simulink model "example_main_NDI_f16"  (R2020a)
settings: Solver=ode4  StartTime=0.0  StopTime=75  FixedStep=0.01  RelTol=1e-3
PreLoadFcn:
  | PreLoadFcn
values from neighbouring files (symbols this model uses):
  g = 32.17    [PreLoadFcn.m]
  N = [ 1      0     0.25 ... (first row only)    [PreLoadFcn.m]
  state0 = [IC.npos IC.epos IC.alt IC.q0 IC.q1 IC.q2 IC.q3  IC.p IC.q IC.r IC.alpha IC.beta IC.mu IC.Vt IC.chi IC.gamma]    [PreLoadFcn.m]
undefined symbols (not defined in the file or in its folder): Aactuator, ac, AeroCoeff, EngineTable, ft, IC, kg, m, Newton, PIController, Raphson, s, sigbuilder_block, slug
libraries: aerolibconvert2 x19, simulink x13, sharedutil x1
(part 4 of 6)

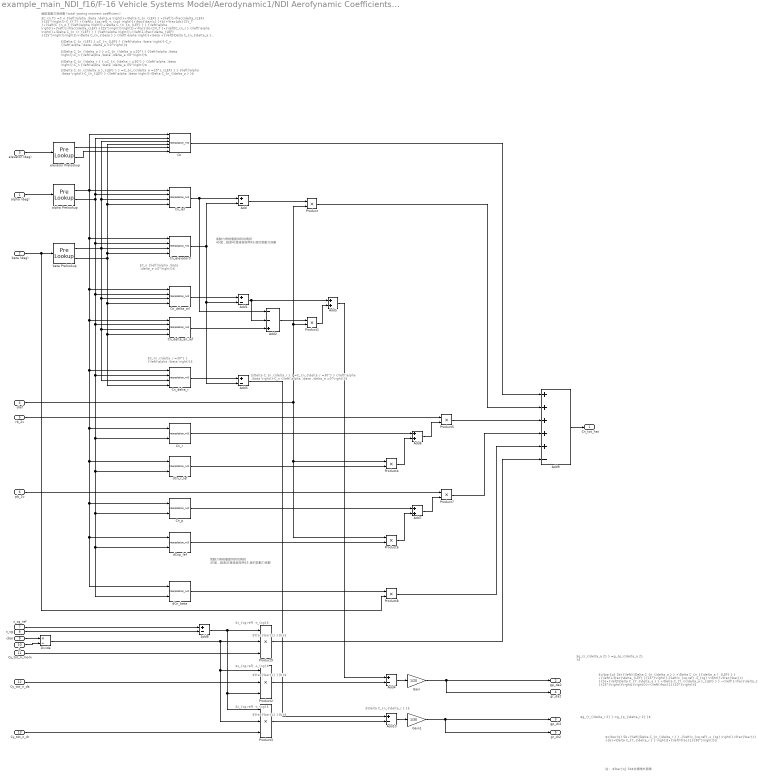
== system example_main_NDI_f16/F-16 Vehicle Systems Model/Aerodynamic1/NDI Aerofynamic Coefficients/CnT ==
  note: $C_n {\left(\alpha ,\beta ,\delta_e =0°\right)}$
  note: $C_{n_{\delta_r =30°} } {\left(\alpha ,\beta \right)}$
  note: $\Delta C_{n_{\delta_r } } =C_{n_{\delta_r =30°} } {\left(\alpha ,\beta \right)}-C_n {\left(\alpha ,\beta ,\delta_e =0°\right)}$
  note: $\Delta C_{n_{\delta_r } }$
  note: $\frac{\bar{c} }{b}$
  note: $x_{cg,ref} -x_{cg}$
  note: 註： $\bar{q} Sb$ 在模塊外面乘
  note: $=\bar{q} Sb∙{\left\{\Delta C_{n_{\delta_a } } +\Delta C_{n_{{\delta_a }_{LEF} } } ∙{\left(1-\frac{\delta_{LEF} }{25°}\right)}-{\left(x_{cg,ref} -x_{cg} \right)}∙\frac{\bar{c} }{b}∙{\left[\Delta C_{Y_{\delta_a } } +\Delta C_{Y_{{\delta_a }_{LEF} } } ∙{\left(1-\frac{\delta_{LEF} }{25°}\right)}\right]}\right\}}∙{\left(\frac{1}{20°}\right)}$
  note: $g_{r_{\delta_a 2} } =g_{p_{\delta_a 2} }$
  note: $=\bar{q} Sb∙{\left[\Delta C_{n_{\delta_r } } -{\left(x_{cg,ref} -x_{cg} \right)}∙\frac{\bar{c} }{b}∙\Delta C_{Y_{\delta_r } } \right]}∙{\left(\frac{1}{30°}\right)}$
  note: $g_{r_{\delta_r 2} } =g_{p_{\delta_r 2} }$
  note: 氣動力表格僅提供到攻角到
      | 45度，超過45度後皆採用45
      | 度的氣動力係數
  note: 氣動力表格僅提供到攻角到
      | 45度，超過45度後皆採用45
      | 度的氣動力係數
  note: $x_{cg,ref} -x_{cg}$
  note: $x_{cg,ref} -x_{cg}$
  note: $\frac{\bar{c} }{b}$
  note: $\frac{\bar{c} }{b}$
  note: $\Delta C_{n_{LEF} } =C_{n_{LEF} } {\left(\alpha ,\beta \right)}-C_n {\left(\alpha ,\beta ,\delta_e =0°\right)}$
  note: 偏航氣動力矩係數 (total yawing moment coefficient)：
  note: $\Delta C_{n_{\delta_a } } =C_{n_{\delta_a =20°} } {\left(\alpha ,\beta \right)}-C_n {\left(\alpha ,\beta ,\delta_e =0°\right)}$
  note: $\Delta C_{n_{\delta_r } } =C_{n_{\delta_r =30°} } {\left(\alpha ,\beta \right)}-C_n {\left(\alpha ,\beta ,\delta_e =0°\right)}$
  note: $\Delta C_{n_{{\delta_a }_{LEF} } } =C_{n_{{\delta_a =20°}_{LEF} } } {\left(\alpha ,\beta \right)}-C_{n_{LEF} } {\left(\alpha ,\beta \right)}-\Delta C_{n_{\delta_a } }$
  note: $C_{n,T} =C_n {\left(\alpha ,\beta ,\delta_e \right)}+\Delta C_{n_{LEF} } ∙{\left(1-\frac{\delta_{LEF} }{25°}\right)}-C_{Y,T} ∙{\left(x_{cg,ref} -x_{cg} \right)}∙\frac{\bar{c} }{b}+\frac{pb}{2V_T }∙{\left[C_{n_p } {\left(\alpha \right)}+\Delta C_{n_{p_{LEF} } } {\left(\alpha \right)}∙{\left(1-\frac{\delta_{LEF} }{25°}\right)}\right]}+\frac{rb}{2V_T }∙{\left[C_{n_r } {\left(\alpha \right)}+\Delta C_{n_{r_{LEF} } } {\left(\alpha \right)}∙{\left(1-\frac{\delta_{LEF} }{25°}\right)}\right]}+\Delta C_{n_{\beta } } {\left(\alpha \right)}∙\beta +{\left[\Delta C_{n_{\delta_a } } +\Delta C_{n_{{\delta_a }_{LEF} } } ∙{\left(1-\frac{\delta_{LEF} }{25°}\right)}\right]}∙{\left(\frac{\delta_a }{20°}\right)}+\Delta C_{n_{\delta_r } } ∙{\left(\frac{\delta_r }{30°}\right)}$
  alpha (deg) : Inport
  beta (deg) : Inport  Port=2
  elevator (deg) : Inport  Port=3
  dlef : Inport  Port=4
  rb_2v : Inport  Port=5
  pb_2v : Inport  Port=6
  x_cg_ref : Inport  Port=7
  x_cg : Inport  Port=8
  cbar : Inport  Port=9
  b : Inport  Port=10
  Cy_tot_n_mom : Inport  Port=11
  Cy_tot_n_da : Inport  Port=12
  Cy_tot_n_dr : Inport  Port=13
  Add{,1,3..4,8,10} (6 alike) : Sum  Inputs=+-
  Add2 : Sum  Inputs=--+
  Add5 : Sum
  Add6 : Sum
  Add7 : Sum
  Add9 : Sum  Inputs=+++++-
  Cn : Interpolation_n-D  NumberOfTableDimensions=3  Table=AeroCoeff.Cn
      settings: InputPortMap=u0,u1,u2,u3,u4,u5
  Cn_delta_ail : Interpolation_n-D  Table=AeroCoeff.Cn_delta_ail
  Cn_delta_ail_lef : Interpolation_n-D  Table=AeroCoeff.Cn_delta_ail_lef
  Cn_delta_r : Interpolation_n-D  Table=AeroCoeff.Cn_delta_r
  Cn_elevator0 : Interpolation_n-D  Table=AeroCoeff.Cn_elevator0
  Cn_lef : Interpolation_n-D  Table=AeroCoeff.Cn_lef
  Cn_p : Interpolation_n-D  NumberOfTableDimensions=1  Table=AeroCoeff.Cn_p
      settings: InputPortMap=u0,u1
  Cn_r : Interpolation_n-D  NumberOfTableDimensions=1  Table=AeroCoeff.Cn_r
      settings: InputPortMap=u0,u1
  Divide : Product  Inputs=*/
  Gain : Gain  Gain=1/20
  Gain1 : Gain  Gain=1/30
  Product{,1,4..8} (7 alike) : Product
  Product2 : Product  Inputs=3
  Product3 : Product  Inputs=3
  Product9 : Product  Inputs=3
  alpha Prelookup : PreLookup  BreakpointsData=AeroCoeff.alpha_prelookup  IndexSearchMethod=Linear search  BeginIndexSearchUsingPreviousIndexResult=on  DiagnosticForOutOfRangeInput=Warning
  beta Prelookup : PreLookup  BreakpointsData=AeroCoeff.beta_prelookup  IndexSearchMethod=Linear search  BeginIndexSearchUsingPreviousIndexResult=on  DiagnosticForOutOfRangeInput=Warning
  dCn_beta : Interpolation_n-D  NumberOfTableDimensions=1  Table=AeroCoeff.dCn_beta
      settings: InputPortMap=u0,u1
  dCn_r_lef : Interpolation_n-D  NumberOfTableDimensions=1  Table=AeroCoeff.dCn_r_lef
      settings: InputPortMap=u0,u1
  dCnp_lef : Interpolation_n-D  NumberOfTableDimensions=1  Table=AeroCoeff.dCnp_lef
      settings: InputPortMap=u0,u1
  elevator Prelookup : PreLookup  BreakpointsData=AeroCoeff.elevator_prelookup1  IndexSearchMethod=Linear search  BeginIndexSearchUsingPreviousIndexResult=on  DiagnosticForOutOfRangeInput=Warning
  Cn_tot_hat : Outport  VectorParamsAs1DForOutWhenUnconnected=off
  gp_da2 : Outport  Port=2  VectorParamsAs1DForOutWhenUnconnected=off
  gp_dr2 : Outport  Port=3  VectorParamsAs1DForOutWhenUnconnected=off
  gr_da2 : Outport  Port=4  VectorParamsAs1DForOutWhenUnconnected=off
  gr_dr2 : Outport  Port=5  VectorParamsAs1DForOutWhenUnconnected=off
  wires:
  alpha Prelookup/1 -> Cn_r/1, dCn_beta/1, dCnp_lef/1, Cn_p/1, dCn_r_lef/1, Cn_delta_r/1, Cn_delta_ail_lef/1, Cn_delta_ail/1, Cn_elevator0/1, Cn/1, Cn_lef/1
  Add8/1 -> Product3/1, Product2/3, Product9/1
  Add1/1 -> Add2/2, Add5/1
  Cn_elevator0/1 -> Add/2, Add3/2, Add1/2
  alpha Prelookup/2 -> Cn_r/2, dCn_beta/2, dCnp_lef/2, Cn_p/2, dCn_r_lef/2, Cn_delta_r/2, Cn_delta_ail_lef/2, Cn_delta_ail/2, Cn_elevator0/2, Cn/2, Cn_lef/2
  elevator Prelookup/1 -> Cn/5
  Add6/1 -> Product5/2
  beta Prelookup/2 -> Cn/4, Cn_lef/4, Cn_elevator0/4, Cn_delta_r/4, Cn_delta_ail_lef/4, Cn_delta_ail/4
  Cn_r/1 -> Add6/1
  Cn_delta_ail_lef/1 -> Add2/3
  pb_2v/1 -> Product7/1
  Cn_lef/1 -> Add2/1, Add/1
  Add7/1 -> Product7/2
  beta (deg)/1 -> beta Prelookup/1, Product8/2
  rb_2v/1 -> Product5/1
  Add/1 -> Product/1
  x_cg/1 -> Add8/2
  alpha (deg)/1 -> alpha Prelookup/1
  b/1 -> Divide/2
  dCn_r_lef/1 -> Product4/2
  dCn_beta/1 -> Product8/1
  Product4/1 -> Add6/2
  Divide/1 -> Product3/2, Product2/1, Product9/2
  x_cg_ref/1 -> Add8/1
  Cn_p/1 -> Add7/1
  dCnp_lef/1 -> Product6/2
  Product8/1 -> Add9/5
  elevator Prelookup/2 -> Cn/6
  Cn_delta_r/1 -> Add3/1
  Product6/1 -> Add7/2
  Cy_tot_n_mom/1 -> Product9/3
  Product7/1 -> Add9/4
  Product5/1 -> Add9/3
  Add2/1 -> Product1/1
  beta Prelookup/1 -> Cn/3, Cn_lef/3, Cn_delta_r/3, Cn_delta_ail_lef/3, Cn_delta_ail/3, Cn_elevator0/3
  Cn/1 -> Add9/1
  Cn_delta_ail/1 -> Add1/1
  Add3/1 -> Add10/1
  elevator (deg)/1 -> elevator Prelookup/1
  dlef/1 -> Product4/1, Product6/1, Product/2, Product1/2
  Product/1 -> Add9/2
  Product1/1 -> Add5/2
  cbar/1 -> Divide/1
  Product9/1 -> Add9/6
  Cy_tot_n_da/1 -> Product2/2
  Product2/1 -> Add4/2
  Add5/1 -> Add4/1
  Add4/1 -> Gain/1
  Cy_tot_n_dr/1 -> Product3/3
  Product3/1 -> Add10/2
  Add10/1 -> Gain1/1
  Add9/1 -> Cn_tot_hat/1
  Gain/1 -> gr_da2/1, gp_da2/1
  Gain1/1 -> gr_dr2/1, gp_dr2/1

== system example_main_NDI_f16/F-16 Vehicle Systems Model/Aerodynamic1/NDI Aerofynamic Coefficients/Ground Effects ==
  alpha (deg) : Inport
  beta(deg) : Inport  Port=2
  h_AGL : Inport  Port=3
  Coeff : Outport

== system example_main_NDI_f16/F-16 Vehicle Systems Model/Aerodynamic1/NDI Aerofynamic Coefficients/Landing Gear Effects ==
  alpha (deg) : Inport
  beta(deg) : Inport  Port=2
  Landing Gear Angle : Inport  Port=3
  Coeff : Outport

== system example_main_NDI_f16/F-16 Vehicle Systems Model/Aerodynamic2/NDI Aerofynamic Coefficients/CXT ==
  note: 氣動力表格僅提供到攻角到
      | 45度，超過45度後皆採用45
      | 度的氣動力係數
  note: $\Delta C_{X_{LEF} } =C_{X_{LEF} } {\left(\alpha ,\beta \right)}-C_X {\left(\alpha ,\beta ,\delta_e =0°\right)}$
  note: $C_{X,T} =C_X {\left(\alpha ,\beta ,\delta_e \right)}+\Delta C_{X_{LEF} } ∙{\left(1-\frac{\delta_{LEF} }{25°}\right)}+\frac{q\bar{c} }{2V_T }∙{\left[C_{X_q } {\left(\alpha \right)}+\Delta C_{X_{q_{LEF} } } {\left(\alpha \right)}∙{\left(1-\frac{\delta_{LEF} }{25°}\right)}\right]}+\Delta C_{X_{SB} } {\left(\alpha \right)}∙{\left(\frac{\delta_{SB} }{60°}\right)}$
  note: 體軸 x 方向之氣動力係數 (total x-axis force coefficient)：
  alpha (deg) : Inport
  beta (deg) : Inport  Port=2
  elevator (deg) : Inport  Port=3
  dlef : Inport  Port=4
  qc_2v : Inport  Port=5
  sb : Inport  Port=6
  Add : Sum  Inputs=+-
  Add1 : Sum  Inputs=++++
  Add2 : Sum
  Cx : Interpolation_n-D  NumberOfTableDimensions=3  Table=AeroCoeff.Cx
      settings: InputPortMap=u0,u1,u2,u3,u4,u5
  Cx_elevator0 : Interpolation_n-D  Table=AeroCoeff.Cx_elevator0
  Cx_lef : Interpolation_n-D  Table=AeroCoeff.Cx_lef
  Cx_q : Interpolation_n-D  NumberOfTableDimensions=1  Table=AeroCoeff.Cx_q
      settings: InputPortMap=u0,u1
  Cx_q_lef : Interpolation_n-D  NumberOfTableDimensions=1  Table=AeroCoeff.Cx_q_lef
      settings: InputPortMap=u0,u1
  Product{,1..3} (4 alike) : Product
  alpha Prelookup : PreLookup  BreakpointsData=AeroCoeff.alpha_prelookup  IndexSearchMethod=Linear search  BeginIndexSearchUsingPreviousIndexResult=on  DiagnosticForOutOfRangeInput=Warning
  beta Prelookup : PreLookup  BreakpointsData=AeroCoeff.beta_prelookup  IndexSearchMethod=Linear search  BeginIndexSearchUsingPreviousIndexResult=on  DiagnosticForOutOfRangeInput=Warning
  dCX_sb : Interpolation_n-D  NumberOfTableDimensions=1  Table=AeroCoeff.dCX_sb
      settings: InputPortMap=u0,u1
  elevator Prelookup : PreLookup  BreakpointsData=AeroCoeff.elevator_prelookup2  IndexSearchMethod=Linear search  BeginIndexSearchUsingPreviousIndexResult=on  DiagnosticForOutOfRangeInput=Warning
  Cx_tot : Outport  VectorParamsAs1DForOutWhenUnconnected=off
  wires:
  beta Prelookup/2 -> Cx_elevator0/4, Cx_lef/4, Cx/4
  alpha (deg)/1 -> alpha Prelookup/1
  beta Prelookup/1 -> Cx_elevator0/3, Cx_lef/3, Cx/3
  Cx_lef/1 -> Add/1
  alpha Prelookup/1 -> Cx_q_lef/1, dCX_sb/1, Cx_q/1, Cx_elevator0/1, Cx/1, Cx_lef/1
  elevator Prelookup/2 -> Cx/6
  elevator (deg)/1 -> elevator Prelookup/1
  beta (deg)/1 -> beta Prelookup/1
  Add/1 -> Product/1
  alpha Prelookup/2 -> Cx_q_lef/2, dCX_sb/2, Cx_q/2, Cx_elevator0/2, Cx_lef/2, Cx/2
  Product/1 -> Add1/2
  elevator Prelookup/1 -> Cx/5
  Add2/1 -> Product2/1
  Cx/1 -> Add1/1
  Cx_elevator0/1 -> Add/2
  Cx_q_lef/1 -> Product1/1
  Product1/1 -> Add2/2
  Cx_q/1 -> Add2/1
  dlef/1 -> Product/2, Product1/2
  Product2/1 -> Add1/3
  Add1/1 -> Cx_tot/1
  qc_2v/1 -> Product2/2
  dCX_sb/1 -> Product3/1
  sb/1 -> Product3/2
  Product3/1 -> Add1/4

== system example_main_NDI_f16/F-16 Vehicle Systems Model/Aerodynamic2/NDI Aerofynamic Coefficients/CYT ==
  note: 氣動力表格僅提供到攻角到
      | 45度，超過45度後皆採用45
      | 度的氣動力係數
  note: 氣動力表格僅提供到攻角到
      | 45度，超過45度後皆採用45
      | 度的氣動力係數
  note: 體軸 y 方向之氣動力係數 (total y-axis force coefficient)：
  note: $\Delta C_{Y_{LEF} }=C_{Y_{LEF} } {\left(\alpha ,\beta \right)}\ \ -C_Y {\left(\alpha ,\beta \right)}$
  note: $\Delta C_{Y_{\delta_r } }=C_{Y_{\delta_r =30°} } {\left(\alpha ,\beta \right)}-C_Y {\left(\alpha ,\beta \right)}$
  note: $C_{Y,T} =C_Y {\left(\alpha ,\beta \right)}+\Delta C_{Y_{LEF} } ∙{\left(1-\frac{\delta_{LEF} }{25°}\right)}+\frac{pb}{2V_T }∙{\left[C_{Y_p } {\left(\alpha \right)}+\Delta C_{{Y_p }_{LEF} } {\left(\alpha \right)}∙{\left(1-\frac{\delta_{LEF} }{25°}\right)}\right]}+\frac{rb}{2V_T }∙{\left[C_{Y_r } {\left(\alpha \right)}+\Delta C_{{Y_r }_{LEF} } {\left(\alpha \right)}∙{\left(1-\frac{\delta_{LEF} }{25°}\right)}\right]}+{\left[\Delta C_{Y_{\delta_a } } +\Delta C_{Y_{{\delta_a }_{LEF} } } ∙{\left(1-\frac{\delta_{LEF} }{25°}\right)}\right]}∙{\left(\frac{\delta_a }{20°}\right)}+\Delta C_{Y_{\delta_r } } ∙{\left(\frac{\delta_r }{30°}\right)}$
  note: $\Delta C_{Y_{{\delta_a }_{LEF} } } =C_{Y_{{\delta_a =20°}_{LEF} } } {\left(\alpha ,\beta \right)}-C_{Y_{LEF} } {\left(\alpha ,\beta \right)}-\Delta C_{Y_{\delta_a } }$
  note: $\Delta C_{Y_{\delta_a } }=C_{Y_{\delta_a =20°} } {\left(\alpha ,\beta \right)}-C_Y {\left(\alpha ,\beta \right)}$
  alpha (deg) : Inport
  beta (deg) : Inport  Port=2
  dlef : Inport  Port=3
  dail : Inport  Port=4
  drud : Inport  Port=5
  rb_2v : Inport  Port=6
  pb_2v : Inport  Port=7
  Add : Sum  Inputs=-+
  Add1 : Sum  Inputs=-+
  Add2 : Sum  Inputs=+--
  Add3 : Sum  Inputs=+-
  Add4 : Sum  Inputs=++++++
  Add5 : Sum
  Add6 : Sum
  Add7 : Sum
  Add8 : Sum  Inputs=++++
  CY : Interpolation_n-D  Table=AeroCoeff.CY
  CY_delta_ail : Interpolation_n-D  Table=AeroCoeff.CY_delta_ail
  CY_delta_ail_lef : Interpolation_n-D  Table=AeroCoeff.CY_delta_ail_lef
  CY_delta_r : Interpolation_n-D  Table=AeroCoeff.CY_delta_r
  CY_lef : Interpolation_n-D  Table=AeroCoeff.CY_lef
  CY_p : Interpolation_n-D  NumberOfTableDimensions=1  Table=AeroCoeff.CY_p
      settings: InputPortMap=u0,u1
  CY_r : Interpolation_n-D  NumberOfTableDimensions=1  Table=AeroCoeff.CY_r
      settings: InputPortMap=u0,u1
  Product{,1..7} (8 alike) : Product
  alpha Prelookup : PreLookup  BreakpointsData=AeroCoeff.alpha_prelookup  IndexSearchMethod=Linear search  BeginIndexSearchUsingPreviousIndexResult=on  DiagnosticForOutOfRangeInput=Warning
  beta Prelookup : PreLookup  BreakpointsData=AeroCoeff.beta_prelookup  IndexSearchMethod=Linear search  BeginIndexSearchUsingPreviousIndexResult=on  DiagnosticForOutOfRangeInput=Warning
  dCY_p_lef : Interpolation_n-D  NumberOfTableDimensions=1  Table=AeroCoeff.dCY_p_lef
      settings: InputPortMap=u0,u1
  dCY_r_lef : Interpolation_n-D  NumberOfTableDimensions=1  Table=AeroCoeff.dCY_r_lef
      settings: InputPortMap=u0,u1
  Cy_tot : Outport  VectorParamsAs1DForOutWhenUnconnected=off
  Cy_tot_n_mom : Outport  Port=2  VectorParamsAs1DForOutWhenUnconnected=off
  Cy_tot_n_da : Outport  Port=3  VectorParamsAs1DForOutWhenUnconnected=off
  Cy_tot_n_dr : Outport  Port=4  VectorParamsAs1DForOutWhenUnconnected=off
  wires:
  Add3/1 -> Cy_tot_n_dr/1, Product3/1
  beta Prelookup/2 -> CY_delta_r/4, CY_delta_ail_lef/4, CY_delta_ail/4, CY/4, CY_lef/4
  beta Prelookup/1 -> CY_delta_r/3, CY_delta_ail_lef/3, CY_delta_ail/3, CY/3, CY_lef/3
  Product7/1 -> Add4/6, Add8/4
  dlef/1 -> Product1/2, Product/2, Product4/2, Product6/1
  alpha Prelookup/1 -> dCY_p_lef/1, CY_p/1, dCY_r_lef/1, CY_r/1, CY_delta_r/1, CY_delta_ail_lef/1, CY_delta_ail/1, CY_lef/1, CY/1
  Add4/1 -> Cy_tot/1
  Add5/1 -> Cy_tot_n_da/1, Product2/1
  CY_p/1 -> Add7/1
  Add1/1 -> Add2/3, Add5/1
  CY_lef/1 -> Add/2, Add2/2
  Add/1 -> Product/1
  dCY_p_lef/1 -> Product6/2
  CY_delta_r/1 -> Add3/1
  CY_delta_ail_lef/1 -> Add2/1
  dCY_r_lef/1 -> Product4/1
  alpha (deg)/1 -> alpha Prelookup/1
  CY_r/1 -> Add6/1
  Product4/1 -> Add6/2
  Add2/1 -> Product1/1
  Product3/1 -> Add4/4
  CY/1 -> Add8/1, Add4/1, Add/1, Add1/1, Add3/2
  Product2/1 -> Add4/3
  Product/1 -> Add4/2, Add8/2
  alpha Prelookup/2 -> CY_p/2, dCY_p_lef/2, dCY_r_lef/2, CY_r/2, CY_delta_r/2, CY_delta_ail_lef/2, CY_delta_ail/2, CY_lef/2, CY/2
  Product6/1 -> Add7/2
  Add6/1 -> Product5/2
  Add7/1 -> Product7/2
  Product5/1 -> Add4/5, Add8/3
  Product1/1 -> Add5/2
  CY_delta_ail/1 -> Add1/2
  beta (deg)/1 -> beta Prelookup/1
  dail/1 -> Product2/2
  drud/1 -> Product3/2
  pb_2v/1 -> Product7/1
  rb_2v/1 -> Product5/1
  Add8/1 -> Cy_tot_n_mom/1

== system example_main_NDI_f16/F-16 Vehicle Systems Model/Aerodynamic2/NDI Aerofynamic Coefficients/CZT ==
  note: CZ
  note: 氣動力表格僅提供到攻角到
      | 45度，超過45度後皆採用45
      | 度的氣動力係數
  note: $\Delta C_{Z_{LEF} } =C_{Z_{LEF} } {\left(\alpha ,\beta \right)}-C_Z {\left(\alpha ,\beta ,\delta_e =0°\right)}$
  note: $C_{Z,T} =C_Z {\left(\alpha ,\beta ,\delta_e \right)}+\Delta C_{Z_{LEF} } ∙{\left(1-\frac{\delta_{LEF} }{25°}\right)}+\frac{q\bar{c} }{2V_T }∙{\left[C_{Z_q } {\left(\alpha \right)}+\Delta C_{Z_{q_{LEF} } } {\left(\alpha \right)}∙{\left(1-\frac{\delta_{LEF} }{25°}\right)}\right]}+\ \Delta C_{Z_{SB} } {\left(\alpha \right)}∙{\left(\frac{\delta_{SB} }{60°}\right)}$
  note: 體軸 z 方向之氣動力係數 (total z-axis force coefficient)：
  alpha (deg) : Inport
  beta (deg) : Inport  Port=2
  elevator (deg) : Inport  Port=3
  dlef : Inport  Port=4
  qc_2v : Inport  Port=5
  sb : Inport  Port=6
  Add : Sum  Inputs=+-
  Add1 : Sum  Inputs=++++
  Add2 : Sum
  Add3 : Sum  Inputs=+++
  Add4 : Sum  Inputs=+++
  Bias : Bias  Bias=0.1
  Bias1 : Bias  Bias=-0.1
  CZ : Interpolation_n-D  NumberOfTableDimensions=3  Table=AeroCoeff.CZ
      settings: InputPortMap=u0,u1,u2,u3,u4,u5
  CZ_elevator0 : Interpolation_n-D  Table=AeroCoeff.CZ_elevator0
  CZ_lef : Interpolation_n-D  Table=AeroCoeff.CZ_lef
  CZ_q : Interpolation_n-D  NumberOfTableDimensions=1  Table=AeroCoeff.CZ_q
      settings: InputPortMap=u0,u1
  Product{,1..3} (4 alike) : Product
  alpha Prelookup : PreLookup  BreakpointsData=AeroCoeff.alpha_prelookup  IndexSearchMethod=Linear search  BeginIndexSearchUsingPreviousIndexResult=on  DiagnosticForOutOfRangeInput=Warning
  beta Prelookup : PreLookup  BreakpointsData=AeroCoeff.beta_prelookup  IndexSearchMethod=Linear search  BeginIndexSearchUsingPreviousIndexResult=on  DiagnosticForOutOfRangeInput=Warning
  dCZ_q_lef : Interpolation_n-D  NumberOfTableDimensions=1  Table=AeroCoeff.dCZ_q_lef
      settings: InputPortMap=u0,u1
  dCZ_sb : Interpolation_n-D  NumberOfTableDimensions=1  Table=AeroCoeff.dCZ_sb
      settings: InputPortMap=u0,u1
  elevator Prelookup : PreLookup  BreakpointsData=AeroCoeff.elevator_prelookup2  IndexSearchMethod=Linear search  BeginIndexSearchUsingPreviousIndexResult=on  DiagnosticForOutOfRangeInput=Warning
  elevator Prelookup1 : PreLookup  BreakpointsData=AeroCoeff.elevator_prelookup2  IndexSearchMethod=Linear search  BeginIndexSearchUsingPreviousIndexResult=on  DiagnosticForOutOfRangeInput=Warning
  elevator Prelookup2 : PreLookup  BreakpointsData=AeroCoeff.elevator_prelookup2  IndexSearchMethod=Linear search  BeginIndexSearchUsingPreviousIndexResult=on  DiagnosticForOutOfRangeInput=Warning
  same as CZ : Interpolation_n-D  NumberOfTableDimensions=3  Table=AeroCoeff.CZ
      settings: InputPortMap=u0,u1,u2,u3,u4,u5
  same_as_CZ : Interpolation_n-D  NumberOfTableDimensions=3  Table=AeroCoeff.CZ
      settings: InputPortMap=u0,u1,u2,u3,u4,u5
  Cz_tot : Outport  VectorParamsAs1DForOutWhenUnconnected=off
  Cz_tot_plus : Outport  Port=2  VectorParamsAs1DForOutWhenUnconnected=off
  Cz_tot_minus : Outport  Port=3  VectorParamsAs1DForOutWhenUnconnected=off
  wires:
  Product2/1 -> Add1/3, Add4/2, Add3/2
  alpha Prelookup/2 -> same as CZ/2, same_as_CZ/2, dCZ_sb/2, dCZ_q_lef/2, CZ_q/2, CZ_elevator0/2, CZ_lef/2, CZ/2
  Add1/1 -> Cz_tot/1
  elevator Prelookup/1 -> CZ/5
  CZ_q/1 -> Add2/1
  beta Prelookup/2 -> same as CZ/4, same_as_CZ/4, CZ_elevator0/4, CZ/4, CZ_lef/4
  CZ_lef/1 -> Add/1
  dCZ_q_lef/1 -> Product1/1
  Product1/1 -> Add2/2
  Add2/1 -> Product2/1
  CZ_elevator0/1 -> Add/2
  Add/1 -> Product/1
  dlef/1 -> Product1/2, Product/2
  Product/1 -> Add3/1, Add4/1, Add1/2
  CZ/1 -> Add1/1
  beta Prelookup/1 -> same as CZ/3, same_as_CZ/3, CZ_elevator0/3, CZ_lef/3, CZ/3
  alpha Prelookup/1 -> same as CZ/1, same_as_CZ/1, dCZ_sb/1, dCZ_q_lef/1, CZ_q/1, CZ_elevator0/1, CZ_lef/1, CZ/1
  alpha (deg)/1 -> alpha Prelookup/1
  elevator Prelookup/2 -> CZ/6
  qc_2v/1 -> Product2/2
  beta (deg)/1 -> beta Prelookup/1
  elevator (deg)/1 -> elevator Prelookup/1, Bias1/1, Bias/1
  Bias/1 -> elevator Prelookup1/1
  Bias1/1 -> elevator Prelookup2/1
  elevator Prelookup1/2 -> same_as_CZ/6
  elevator Prelookup1/1 -> same_as_CZ/5
  elevator Prelookup2/2 -> same as CZ/6
  elevator Prelookup2/1 -> same as CZ/5
  same_as_CZ/1 -> Add3/3
  same as CZ/1 -> Add4/3
  Add3/1 -> Cz_tot_plus/1
  Add4/1 -> Cz_tot_minus/1
  sb/1 -> Product3/2
  dCZ_sb/1 -> Product3/1
  Product3/1 -> Add1/4

== system example_main_NDI_f16/F-16 Vehicle Systems Model/Aerodynamic2/NDI Aerofynamic Coefficients/ClT ==
  note: 氣動力表格僅提供到攻角到
      | 45度，超過45度後皆採用45
      | 度的氣動力係數
  note: 氣動力表格僅提供到攻角到
      | 45度，超過45度後皆採用45
      | 度的氣動力係數
  note: $\Delta C_{l_{LEF} } =C_{l_{LEF} } {\left(\alpha ,\beta \right)}-C_l {\left(\alpha ,\beta ,\delta_e =0°\right)}$
  note: $\Delta C_{l_{\delta_a } } =C_{l_{\delta_a =20°} } {\left(\alpha ,\beta \right)}-C_l {\left(\alpha ,\beta ,\delta_e =0°\right)}$
  note: $C_{l,T} =C_l {\left(\alpha ,\beta ,\delta_e \right)}+\Delta C_{l_{LEF} } ∙{\left(1-\frac{\delta_{LEF} }{25°}\right)}+\frac{pb}{2V_T }∙{\left[C_{l_p } {\left(\alpha \right)}+\Delta C_{l_{p_{LEF} } } {\left(\alpha \right)}∙{\left(1-\frac{\delta_{LEF} }{25°}\right)}+\frac{rb}{2V_T }∙{\left[C_{l_r } {\left(\alpha \right)}+\Delta C_{l_{r_{LEF} } } {\left(\alpha \right)}∙{\left(1-\frac{\delta_{LEF} }{25°}\right)}\right]}+\Delta C_{l_{\beta } } {\left(\alpha \right)}∙\beta +{\left[\Delta C_{l_{\delta_a } } +\Delta C_{l_{{\delta_a }_{LEF} } } ∙{\left(1-\frac{\delta_{LEF} }{25°}\right)}\right]}∙{\left(\frac{\delta_a }{20°}\right)}+\Delta C_{l_{\delta_r } } ∙{\left(\frac{\delta_r }{30°}\right)}\right]}$
  note: 側滾氣動力矩係數 (total rolling moment coefficient)：
  note: $\Delta C_{l_{\delta_r } } =C_{l_{\delta_r =30°} } {\left(\alpha ,\beta \right)}-C_l {\left(\alpha ,\beta ,\delta_e =0°\right)}$
  note: $\Delta C_{l_{{\delta_a }_{LEF} } } =C_{l_{{\delta_a =20°}_{LEF} } } {\left(\alpha ,\beta \right)}-C_{l_{LEF} } {\left(\alpha ,\beta \right)}-\Delta C_{l_{\delta_a } }$
  alpha (deg) : Inport
  beta (deg) : Inport  Port=2
  elevator (deg) : Inport  Port=3
  dlef : Inport  Port=4
  rb_2v : Inport  Port=5
  pb_2v : Inport  Port=6
  Cl : Interpolation_n-D  NumberOfTableDimensions=3  Table=AeroCoeff.Cl
      settings: InputPortMap=u0,u1,u2,u3,u4,u5
  Cl_delta_ail : Interpolation_n-D  Table=AeroCoeff.Cl_delta_ail  InternalRulePriority=Speed
  Cl_delta_ail_lef : Interpolation_n-D  Table=AeroCoeff.Cl_delta_ail_lef  InternalRulePriority=Speed
  Cl_delta_r : Interpolation_n-D  Table=AeroCoeff.Cl_delta_r  InternalRulePriority=Speed
  Cl_elevator0 : Interpolation_n-D  Table=AeroCoeff.Cl_elevator0
  Cl_lef : Interpolation_n-D  Table=AeroCoeff.Cl_lef  InternalRulePriority=Speed
  Cl_p : Interpolation_n-D  NumberOfTableDimensions=1  Table=AeroCoeff.Cl_p  InternalRulePriority=Speed
      settings: InputPortMap=u0,u1
  Cl_r : Interpolation_n-D  NumberOfTableDimensions=1  Table=AeroCoeff.Cl_r  InternalRulePriority=Speed
      settings: InputPortMap=u0,u1
  Gain : Gain  Gain=1/20
  Gain1 : Gain  Gain=1/30
  Product{,1,4..8} (7 alike) : Product
  Subtract : Sum  Inputs=+-
  Subtract1 : Sum  Inputs=+-
  Subtract2 : Sum  Inputs=+--
  Subtract3 : Sum  Inputs=+-
  Subtract5 : Sum
  Subtract6 : Sum
  Subtract7 : Sum
  Subtract8 : Sum  Inputs=+++++
  alpha Prelookup : PreLookup  BreakpointsData=AeroCoeff.alpha_prelookup  IndexSearchMethod=Linear search  BeginIndexSearchUsingPreviousIndexResult=on  DiagnosticForOutOfRangeInput=Warning
  beta Prelookup : PreLookup  BreakpointsData=AeroCoeff.beta_prelookup  IndexSearchMethod=Linear search  BeginIndexSearchUsingPreviousIndexResult=on  DiagnosticForOutOfRangeInput=Warning
  dCl_beta : Interpolation_n-D  NumberOfTableDimensions=1  Table=AeroCoeff.dCl_beta  InternalRulePriority=Speed
      settings: InputPortMap=u0,u1
  dCl_p_lef : Interpolation_n-D  NumberOfTableDimensions=1  Table=AeroCoeff.dCl_p_lef  InternalRulePriority=Speed
      settings: InputPortMap=u0,u1
  dCl_r_lef : Interpolation_n-D  NumberOfTableDimensions=1  Table=AeroCoeff.dCl_r_lef  InternalRulePriority=Speed
      settings: InputPortMap=u0,u1
  elevator Prelookup : PreLookup  BreakpointsData=AeroCoeff.elevator_prelookup1  IndexSearchMethod=Linear search  BeginIndexSearchUsingPreviousIndexResult=on  DiagnosticForOutOfRangeInput=Warning
  Cl_tot_hat : Outport  VectorParamsAs1DForOutWhenUnconnected=off
  gp_da1 : Outport  Port=2  VectorParamsAs1DForOutWhenUnconnected=off
  gp_dr1 : Outport  Port=3  VectorParamsAs1DForOutWhenUnconnected=off
  gr_da1 : Outport  Port=4  VectorParamsAs1DForOutWhenUnconnected=off
  gr_dr1 : Outport  Port=5  VectorParamsAs1DForOutWhenUnconnected=off
  wires:
  Cl_elevator0/1 -> Subtract3/2, Subtract1/2, Subtract/2
  beta Prelookup/1 -> Cl/3, Cl_lef/3, Cl_elevator0/3, Cl_delta_ail_lef/3, Cl_delta_r/3, Cl_delta_ail/3
  Cl_delta_r/1 -> Subtract3/1
  Cl_lef/1 -> Subtract2/2, Subtract/1
  Subtract/1 -> Product/1
  Product6/1 -> Subtract7/2
  alpha Prelookup/1 -> dCl_r_lef/1, dCl_p_lef/1, dCl_beta/1, Cl_p/1, Cl_r/1, Cl_delta_r/1, Cl_delta_ail_lef/1, Cl_delta_ail/1, Cl_elevator0/1, Cl/1, Cl_lef/1
  Cl_p/1 -> Subtract7/1
  beta (deg)/1 -> beta Prelookup/1, Product8/2
  Subtract2/1 -> Product1/1
  alpha Prelookup/2 -> Cl_r/2, dCl_r_lef/2, dCl_p_lef/2, dCl_beta/2, Cl_p/2, Cl_delta_r/2, Cl_delta_ail_lef/2, Cl_delta_ail/2, Cl/2, Cl_lef/2, Cl_elevator0/2
  alpha (deg)/1 -> alpha Prelookup/1
  Product/1 -> Subtract8/2
  Subtract6/1 -> Product5/2
  rb_2v/1 -> Product5/1
  Cl_delta_ail/1 -> Subtract1/1
  elevator Prelookup/1 -> Cl/5
  Product7/1 -> Subtract8/4
  Subtract7/1 -> Product7/1
  Product5/1 -> Subtract8/3
  dCl_r_lef/1 -> Product4/1
  Subtract3/1 -> Gain1/1
  Subtract1/1 -> Subtract2/3, Subtract5/1
  dlef/1 -> Product6/1, Product4/2, Product/2, Product1/2
  Cl_delta_ail_lef/1 -> Subtract2/1
  beta Prelookup/2 -> Cl/4, Cl_lef/4, Cl_elevator0/4, Cl_delta_ail/4, Cl_delta_ail_lef/4, Cl_delta_r/4
  Product4/1 -> Subtract6/2
  dCl_beta/1 -> Product8/1
  Product1/1 -> Subtract5/2
  dCl_p_lef/1 -> Product6/2
  Product8/1 -> Subtract8/5
  Cl_r/1 -> Subtract6/1
  elevator Prelookup/2 -> Cl/6
  Cl/1 -> Subtract8/1
  pb_2v/1 -> Product7/2
  elevator (deg)/1 -> elevator Prelookup/1
  Subtract8/1 -> Cl_tot_hat/1
  Subtract5/1 -> Gain/1
  Gain/1 -> gp_da1/1, gr_da1/1
  Gain1/1 -> gp_dr1/1, gr_dr1/1

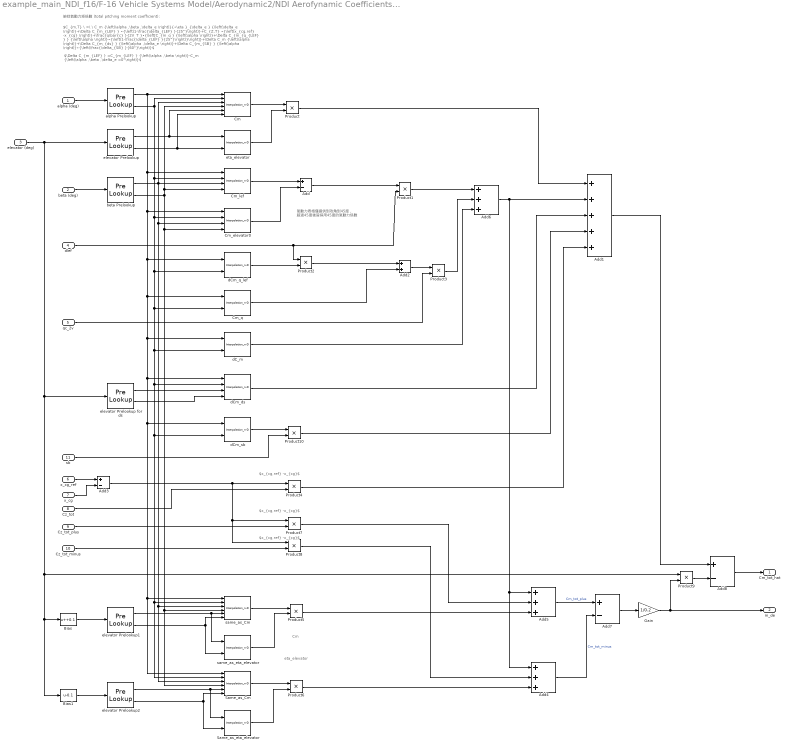
== system example_main_NDI_f16/F-16 Vehicle Systems Model/Aerodynamic2/NDI Aerofynamic Coefficients/CmT ==
  note: $x_{cg,ref} -x_{cg}$
  note: eta_elevator
  note: Cm
  note: 氣動力表格僅提供到攻角到45度，
      | 超過45度後皆採用45度的氣動力係數
  note: $x_{cg,ref} -x_{cg}$
  note: $x_{cg,ref} -x_{cg}$
  note: $C_{m,T} \ =\ \ C_m {\left(\alpha ,\beta ,\delta_e \right)}{∙\eta }_{\delta_e } {\left(\delta_e \right)}+\Delta C_{m_{LEF} } ∙{\left(1-\frac{\delta_{LEF} }{25°}\right)}+C_{Z,T} ∙{\left(x_{cg,ref} -x_{cg} \right)}+\frac{q\bar{c} }{2V_T }∙{\left[C_{m_q } {\left(\alpha \right)}+\Delta C_{m_{q_{LEF} } } {\left(\alpha \right)}∙{\left(1-\frac{\delta_{LEF} }{25°}\right)}\right]}+\Delta C_m {\left(\alpha \right)}+\Delta C_{m_{ds} } {\left(\alpha ,\delta_e \right)}+\Delta C_{m_{SB} } {\left(\alpha \right)}∙{\left(\frac{\delta_{SB} }{60°}\right)}$
  note: $\Delta C_{m_{LEF} } =C_{m_{LEF} } {\left(\alpha ,\beta \right)}-C_m {\left(\alpha ,\beta ,\delta_e =0°\right)}$
  note: 俯仰氣動力矩係數 (total pitching moment coefficient)：
  alpha (deg) : Inport
  beta (deg) : Inport  Port=2
  elevator (deg) : Inport  Port=3
  dlef : Inport  Port=4
  qc_2v : Inport  Port=5
  x_cg_ref : Inport  Port=6
  x_cg : Inport  Port=7
  Cz_tot : Inport  Port=8
  Cz_tot_plus : Inport  Port=9
  Cz_tot_minus : Inport  Port=10
  sb : Inport  Port=11
  Add{,3,7..8} (4 alike) : Sum  Inputs=+-
  Add1 : Sum  Inputs=+++++
  Add2 : Sum
  Add4 : Sum  Inputs=+++
  Add5 : Sum  Inputs=+++
  Add6 : Sum  Inputs=+++
  Bias : Bias  Bias=+0.1
  Bias1 : Bias  Bias=-0.1
  Cm : Interpolation_n-D  NumberOfTableDimensions=3  Table=AeroCoeff.Cm
      settings: InputPortMap=u0,u1,u2,u3,u4,u5
  Cm_elevator0 : Interpolation_n-D  Table=AeroCoeff.Cm_elevator0
  Cm_lef : Interpolation_n-D  Table=AeroCoeff.Cm_lef
  Cm_q : Interpolation_n-D  NumberOfTableDimensions=1  Table=AeroCoeff.Cm_q
      settings: InputPortMap=u0,u1
  Gain : Gain  Gain=1/0.2
  Product{,1..10} (11 alike) : Product
  Same_as_Cm : Interpolation_n-D  NumberOfTableDimensions=3  Table=AeroCoeff.Cm
      settings: InputPortMap=u0,u1,u2,u3,u4,u5
  Same_as_eta_elevator : Interpolation_n-D  NumberOfTableDimensions=1  Table=AeroCoeff.eta_elevator
      settings: InputPortMap=u0,u1
  alpha Prelookup : PreLookup  BreakpointsData=AeroCoeff.alpha_prelookup  IndexSearchMethod=Linear search  BeginIndexSearchUsingPreviousIndexResult=on  DiagnosticForOutOfRangeInput=Warning
  beta Prelookup : PreLookup  BreakpointsData=AeroCoeff.beta_prelookup  IndexSearchMethod=Linear search  BeginIndexSearchUsingPreviousIndexResult=on  DiagnosticForOutOfRangeInput=Warning
  dC_m : Interpolation_n-D  NumberOfTableDimensions=1  Table=AeroCoeff.dC_m
      settings: InputPortMap=u0,u1
  dCm_ds : Interpolation_n-D  Table=AeroCoeff.dCm_ds
  dCm_q_lef : Interpolation_n-D  NumberOfTableDimensions=1  Table=AeroCoeff.dCm_q_lef
      settings: InputPortMap=u0,u1
  dCm_sb : Interpolation_n-D  NumberOfTableDimensions=1  Table=AeroCoeff.dCm_sb
      settings: InputPortMap=u0,u1
  elevator Prelookup : PreLookup  BreakpointsData=AeroCoeff.elevator_prelookup2  IndexSearchMethod=Linear search  BeginIndexSearchUsingPreviousIndexResult=on  DiagnosticForOutOfRangeInput=Warning
  elevator Prelookup for ds : PreLookup  BreakpointsData=AeroCoeff.elevator_prelookup3  IndexSearchMethod=Linear search  BeginIndexSearchUsingPreviousIndexResult=on  DiagnosticForOutOfRangeInput=Warning
  elevator Prelookup1 : PreLookup  BreakpointsData=AeroCoeff.elevator_prelookup2  IndexSearchMethod=Linear search  BeginIndexSearchUsingPreviousIndexResult=on  DiagnosticForOutOfRangeInput=Warning
  elevator Prelookup2 : PreLookup  BreakpointsData=AeroCoeff.elevator_prelookup2  IndexSearchMethod=Linear search  BeginIndexSearchUsingPreviousIndexResult=on  DiagnosticForOutOfRangeInput=Warning
  eta_elevator : Interpolation_n-D  NumberOfTableDimensions=1  Table=AeroCoeff.eta_elevator
      settings: InputPortMap=u0,u1
  same_as_Cm : Interpolation_n-D  NumberOfTableDimensions=3  Table=AeroCoeff.Cm
      settings: InputPortMap=u0,u1,u2,u3,u4,u5
  same_as_eta_elevator : Interpolation_n-D  NumberOfTableDimensions=1  Table=AeroCoeff.eta_elevator
      settings: InputPortMap=u0,u1
  Cm_tot_hat : Outport  VectorParamsAs1DForOutWhenUnconnected=off
  m_de : Outport  Port=2  VectorParamsAs1DForOutWhenUnconnected=off
  wires:
  Cm/1 -> Product/1
  Cm_lef/1 -> Add/1
  Add3/1 -> Product8/1, Product7/1, Product4/1
  Product3/1 -> Add6/2
  alpha Prelookup/1 -> Same_as_Cm/1, same_as_Cm/1, dCm_sb/1, dCm_ds/1, dC_m/1, Cm_q/1, dCm_q_lef/1, Cm_elevator0/1, Cm_lef/1, Cm/1
  Cm_elevator0/1 -> Add/2
  elevator Prelookup/1 -> Cm/5, eta_elevator/1
  dC_m/1 -> Add6/3
  alpha Prelookup/2 -> Cm/2, Same_as_Cm/2, same_as_Cm/2, dCm_sb/2, dCm_ds/2, dC_m/2, Cm_q/2, dCm_q_lef/2, Cm_elevator0/2, Cm_lef/2
  dlef/1 -> Product2/1, Product1/2
  elevator Prelookup/2 -> Cm/6, eta_elevator/2
  elevator (deg)/1 -> elevator Prelookup/1, Bias1/1, Bias/1, Product9/1, elevator Prelookup for ds/1
  Product1/1 -> Add6/1
  eta_elevator/1 -> Product/2
  beta Prelookup/2 -> Same_as_Cm/4, same_as_Cm/4, Cm_elevator0/4, Cm/4, Cm_lef/4
  Product2/1 -> Add2/1
  Cm_q/1 -> Add2/2
  beta Prelookup/1 -> Cm/3, Same_as_Cm/3, same_as_Cm/3, Cm_elevator0/3, Cm_lef/3
  Product/1 -> Add1/1
  dCm_q_lef/1 -> Product2/2
  Add2/1 -> Product3/1
  Add/1 -> Product1/1
  qc_2v/1 -> Product3/2
  alpha (deg)/1 -> alpha Prelookup/1
  Product4/1 -> Add1/5
  beta (deg)/1 -> beta Prelookup/1
  x_cg/1 -> Add3/2
  Add1/1 -> Add8/1
  Cz_tot/1 -> Product4/2
  x_cg_ref/1 -> Add3/1
  Bias/1 -> elevator Prelookup1/1
  Bias1/1 -> elevator Prelookup2/1
  elevator Prelookup1/1 -> same_as_Cm/5, same_as_eta_elevator/1
  elevator Prelookup1/2 -> same_as_Cm/6, same_as_eta_elevator/2
  elevator Prelookup2/1 -> Same_as_eta_elevator/1, Same_as_Cm/5
  elevator Prelookup2/2 -> Same_as_Cm/6, Same_as_eta_elevator/2
  same_as_Cm/1 -> Product5/1
  same_as_eta_elevator/1 -> Product5/2
  Same_as_Cm/1 -> Product6/1
  Same_as_eta_elevator/1 -> Product6/2
  Product5/1 -> Add5/3
  Cz_tot_plus/1 -> Product7/2
  Cz_tot_minus/1 -> Product8/2
  Product7/1 -> Add5/2
  Product6/1 -> Add4/3
  Product8/1 -> Add4/2
  Add6/1 -> Add1/2, Add4/1, Add5/1
  Add5/1 -> Add7/1  "Cm_tot_plus"
  Add4/1 -> Add7/2  "Cm_tot_minus"
  Add7/1 -> Gain/1
  Gain/1 -> m_de/1, Product9/2
  Product9/1 -> Add8/2
  Add8/1 -> Cm_tot_hat/1
  sb/1 -> Product10/2
  dCm_sb/1 -> Product10/1
  Product10/1 -> Add1/4
  elevator Prelookup for ds/1 -> dCm_ds/3
  elevator Prelookup for ds/2 -> dCm_ds/4
  dCm_ds/1 -> Add1/3

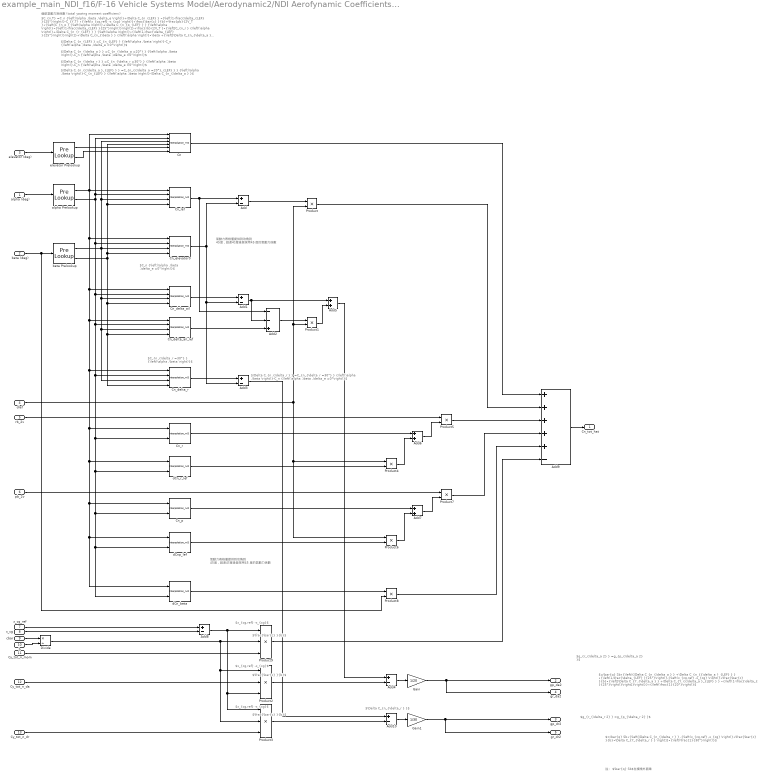
== system example_main_NDI_f16/F-16 Vehicle Systems Model/Aerodynamic2/NDI Aerofynamic Coefficients/CnT ==
  note: $C_n {\left(\alpha ,\beta ,\delta_e =0°\right)}$
  note: $C_{n_{\delta_r =30°} } {\left(\alpha ,\beta \right)}$
  note: $\Delta C_{n_{\delta_r } } =C_{n_{\delta_r =30°} } {\left(\alpha ,\beta \right)}-C_n {\left(\alpha ,\beta ,\delta_e =0°\right)}$
  note: $\Delta C_{n_{\delta_r } }$
  note: $\frac{\bar{c} }{b}$
  note: $x_{cg,ref} -x_{cg}$
  note: 註： $\bar{q} Sb$ 在模塊外面乘
  note: $=\bar{q} Sb∙{\left\{\Delta C_{n_{\delta_a } } +\Delta C_{n_{{\delta_a }_{LEF} } } ∙{\left(1-\frac{\delta_{LEF} }{25°}\right)}-{\left(x_{cg,ref} -x_{cg} \right)}∙\frac{\bar{c} }{b}∙{\left[\Delta C_{Y_{\delta_a } } +\Delta C_{Y_{{\delta_a }_{LEF} } } ∙{\left(1-\frac{\delta_{LEF} }{25°}\right)}\right]}\right\}}∙{\left(\frac{1}{20°}\right)}$
  note: $g_{r_{\delta_a 2} } =g_{p_{\delta_a 2} }$
  note: $=\bar{q} Sb∙{\left[\Delta C_{n_{\delta_r } } -{\left(x_{cg,ref} -x_{cg} \right)}∙\frac{\bar{c} }{b}∙\Delta C_{Y_{\delta_r } } \right]}∙{\left(\frac{1}{30°}\right)}$
  note: $g_{r_{\delta_r 2} } =g_{p_{\delta_r 2} }$
  note: 氣動力表格僅提供到攻角到
      | 45度，超過45度後皆採用45
      | 度的氣動力係數
  note: 氣動力表格僅提供到攻角到
      | 45度，超過45度後皆採用45
      | 度的氣動力係數
  note: $x_{cg,ref} -x_{cg}$
  note: $x_{cg,ref} -x_{cg}$
  note: $\frac{\bar{c} }{b}$
  note: $\frac{\bar{c} }{b}$
  note: $\Delta C_{n_{LEF} } =C_{n_{LEF} } {\left(\alpha ,\beta \right)}-C_n {\left(\alpha ,\beta ,\delta_e =0°\right)}$
  note: 偏航氣動力矩係數 (total yawing moment coefficient)：
  note: $\Delta C_{n_{\delta_a } } =C_{n_{\delta_a =20°} } {\left(\alpha ,\beta \right)}-C_n {\left(\alpha ,\beta ,\delta_e =0°\right)}$
  note: $\Delta C_{n_{\delta_r } } =C_{n_{\delta_r =30°} } {\left(\alpha ,\beta \right)}-C_n {\left(\alpha ,\beta ,\delta_e =0°\right)}$
  note: $\Delta C_{n_{{\delta_a }_{LEF} } } =C_{n_{{\delta_a =20°}_{LEF} } } {\left(\alpha ,\beta \right)}-C_{n_{LEF} } {\left(\alpha ,\beta \right)}-\Delta C_{n_{\delta_a } }$
  note: $C_{n,T} =C_n {\left(\alpha ,\beta ,\delta_e \right)}+\Delta C_{n_{LEF} } ∙{\left(1-\frac{\delta_{LEF} }{25°}\right)}-C_{Y,T} ∙{\left(x_{cg,ref} -x_{cg} \right)}∙\frac{\bar{c} }{b}+\frac{pb}{2V_T }∙{\left[C_{n_p } {\left(\alpha \right)}+\Delta C_{n_{p_{LEF} } } {\left(\alpha \right)}∙{\left(1-\frac{\delta_{LEF} }{25°}\right)}\right]}+\frac{rb}{2V_T }∙{\left[C_{n_r } {\left(\alpha \right)}+\Delta C_{n_{r_{LEF} } } {\left(\alpha \right)}∙{\left(1-\frac{\delta_{LEF} }{25°}\right)}\right]}+\Delta C_{n_{\beta } } {\left(\alpha \right)}∙\beta +{\left[\Delta C_{n_{\delta_a } } +\Delta C_{n_{{\delta_a }_{LEF} } } ∙{\left(1-\frac{\delta_{LEF} }{25°}\right)}\right]}∙{\left(\frac{\delta_a }{20°}\right)}+\Delta C_{n_{\delta_r } } ∙{\left(\frac{\delta_r }{30°}\right)}$
  alpha (deg) : Inport
  beta (deg) : Inport  Port=2
  elevator (deg) : Inport  Port=3
  dlef : Inport  Port=4
  rb_2v : Inport  Port=5
  pb_2v : Inport  Port=6
  x_cg_ref : Inport  Port=7
  x_cg : Inport  Port=8
  cbar : Inport  Port=9
  b : Inport  Port=10
  Cy_tot_n_mom : Inport  Port=11
  Cy_tot_n_da : Inport  Port=12
  Cy_tot_n_dr : Inport  Port=13
  Add{,1,3..4,8,10} (6 alike) : Sum  Inputs=+-
  Add2 : Sum  Inputs=--+
  Add5 : Sum
  Add6 : Sum
  Add7 : Sum
  Add9 : Sum  Inputs=+++++-
  Cn : Interpolation_n-D  NumberOfTableDimensions=3  Table=AeroCoeff.Cn
      settings: InputPortMap=u0,u1,u2,u3,u4,u5
  Cn_delta_ail : Interpolation_n-D  Table=AeroCoeff.Cn_delta_ail
  Cn_delta_ail_lef : Interpolation_n-D  Table=AeroCoeff.Cn_delta_ail_lef
  Cn_delta_r : Interpolation_n-D  Table=AeroCoeff.Cn_delta_r
  Cn_elevator0 : Interpolation_n-D  Table=AeroCoeff.Cn_elevator0
  Cn_lef : Interpolation_n-D  Table=AeroCoeff.Cn_lef
  Cn_p : Interpolation_n-D  NumberOfTableDimensions=1  Table=AeroCoeff.Cn_p
      settings: InputPortMap=u0,u1
  Cn_r : Interpolation_n-D  NumberOfTableDimensions=1  Table=AeroCoeff.Cn_r
      settings: InputPortMap=u0,u1
  Divide : Product  Inputs=*/
  Gain : Gain  Gain=1/20
  Gain1 : Gain  Gain=1/30
  Product{,1,4..8} (7 alike) : Product
  Product2 : Product  Inputs=3
  Product3 : Product  Inputs=3
  Product9 : Product  Inputs=3
  alpha Prelookup : PreLookup  BreakpointsData=AeroCoeff.alpha_prelookup  IndexSearchMethod=Linear search  BeginIndexSearchUsingPreviousIndexResult=on  DiagnosticForOutOfRangeInput=Warning
  beta Prelookup : PreLookup  BreakpointsData=AeroCoeff.beta_prelookup  IndexSearchMethod=Linear search  BeginIndexSearchUsingPreviousIndexResult=on  DiagnosticForOutOfRangeInput=Warning
  dCn_beta : Interpolation_n-D  NumberOfTableDimensions=1  Table=AeroCoeff.dCn_beta
      settings: InputPortMap=u0,u1
  dCn_r_lef : Interpolation_n-D  NumberOfTableDimensions=1  Table=AeroCoeff.dCn_r_lef
      settings: InputPortMap=u0,u1
  dCnp_lef : Interpolation_n-D  NumberOfTableDimensions=1  Table=AeroCoeff.dCnp_lef
      settings: InputPortMap=u0,u1
  elevator Prelookup : PreLookup  BreakpointsData=AeroCoeff.elevator_prelookup1  IndexSearchMethod=Linear search  BeginIndexSearchUsingPreviousIndexResult=on  DiagnosticForOutOfRangeInput=Warning
  Cn_tot_hat : Outport  VectorParamsAs1DForOutWhenUnconnected=off
  gp_da2 : Outport  Port=2  VectorParamsAs1DForOutWhenUnconnected=off
  gp_dr2 : Outport  Port=3  VectorParamsAs1DForOutWhenUnconnected=off
  gr_da2 : Outport  Port=4  VectorParamsAs1DForOutWhenUnconnected=off
  gr_dr2 : Outport  Port=5  VectorParamsAs1DForOutWhenUnconnected=off
  wires:
  alpha Prelookup/1 -> Cn_r/1, dCn_beta/1, dCnp_lef/1, Cn_p/1, dCn_r_lef/1, Cn_delta_r/1, Cn_delta_ail_lef/1, Cn_delta_ail/1, Cn_elevator0/1, Cn/1, Cn_lef/1
  Add8/1 -> Product3/1, Product2/3, Product9/1
  Add1/1 -> Add2/2, Add5/1
  Cn_elevator0/1 -> Add/2, Add3/2, Add1/2
  alpha Prelookup/2 -> Cn_r/2, dCn_beta/2, dCnp_lef/2, Cn_p/2, dCn_r_lef/2, Cn_delta_r/2, Cn_delta_ail_lef/2, Cn_delta_ail/2, Cn_elevator0/2, Cn/2, Cn_lef/2
  elevator Prelookup/1 -> Cn/5
  Add6/1 -> Product5/2
  beta Prelookup/2 -> Cn/4, Cn_lef/4, Cn_elevator0/4, Cn_delta_r/4, Cn_delta_ail_lef/4, Cn_delta_ail/4
  Cn_r/1 -> Add6/1
  Cn_delta_ail_lef/1 -> Add2/3
  pb_2v/1 -> Product7/1
  Cn_lef/1 -> Add2/1, Add/1
  Add7/1 -> Product7/2
  beta (deg)/1 -> beta Prelookup/1, Product8/2
  rb_2v/1 -> Product5/1
  Add/1 -> Product/1
  x_cg/1 -> Add8/2
  alpha (deg)/1 -> alpha Prelookup/1
  b/1 -> Divide/2
  dCn_r_lef/1 -> Product4/2
  dCn_beta/1 -> Product8/1
  Product4/1 -> Add6/2
  Divide/1 -> Product3/2, Product2/1, Product9/2
  x_cg_ref/1 -> Add8/1
  Cn_p/1 -> Add7/1
  dCnp_lef/1 -> Product6/2
  Product8/1 -> Add9/5
  elevator Prelookup/2 -> Cn/6
  Cn_delta_r/1 -> Add3/1
  Product6/1 -> Add7/2
  Cy_tot_n_mom/1 -> Product9/3
  Product7/1 -> Add9/4
  Product5/1 -> Add9/3
  Add2/1 -> Product1/1
  beta Prelookup/1 -> Cn/3, Cn_lef/3, Cn_delta_r/3, Cn_delta_ail_lef/3, Cn_delta_ail/3, Cn_elevator0/3
  Cn/1 -> Add9/1
  Cn_delta_ail/1 -> Add1/1
  Add3/1 -> Add10/1
  elevator (deg)/1 -> elevator Prelookup/1
  dlef/1 -> Product4/1, Product6/1, Product/2, Product1/2
  Product/1 -> Add9/2
  Product1/1 -> Add5/2
  cbar/1 -> Divide/1
  Product9/1 -> Add9/6
  Cy_tot_n_da/1 -> Product2/2
  Product2/1 -> Add4/2
  Add5/1 -> Add4/1
  Add4/1 -> Gain/1
  Cy_tot_n_dr/1 -> Product3/3
  Product3/1 -> Add10/2
  Add10/1 -> Gain1/1
  Add9/1 -> Cn_tot_hat/1
  Gain/1 -> gr_da2/1, gp_da2/1
  Gain1/1 -> gr_dr2/1, gp_dr2/1

== system example_main_NDI_f16/F-16 Vehicle Systems Model/Aerodynamic2/NDI Aerofynamic Coefficients/Ground Effects ==
  alpha (deg) : Inport
  beta(deg) : Inport  Port=2
  h_AGL : Inport  Port=3
  Coeff : Outport

== system example_main_NDI_f16/F-16 Vehicle Systems Model/Aerodynamic2/NDI Aerofynamic Coefficients/Landing Gear Effects ==
  alpha (deg) : Inport
  beta(deg) : Inport  Port=2
  Landing Gear Angle : Inport  Port=3
  Coeff : Outport

== system example_main_NDI_f16/F-16 Vehicle Systems Model/Vehicle/6DOF (Quaternion)/Quaternion Normalization ==
  q : Inport  PortDimensions=4
  Product : Product  Inputs=*/  InputSameDT=on  RndMeth=Zero  SaturateOnIntegerOverflow=on  OutDataTypeStr=Inherit: Same as first input
  Square : Math  Operator=square  SignedPower=on  SaturateOnIntegerOverflow=on
  Square Root : Sqrt  Operator=signedSqrt  AlgorithmType=Newton-Raphson  SaturateOnIntegerOverflow=on
  Sum : Sum  Inputs=1  InputSameDT=on  SaturateOnIntegerOverflow=on  OutDataTypeStr=Inherit: Same as first input
  qnorm : Outport  VectorParamsAs1DForOutWhenUnconnected=off
  wires:
  Product/1 -> qnorm/1
  Square Root/1 -> Product/2
  Square/1 -> Sum/1
  Sum/1 -> Square Root/1
  q/1 -> Product/1, Square/1

== system example_main_NDI_f16/F-16 Vehicle Systems Model/Vehicle/Actuators (no roll off)1/Engine block ==
  Mach : Inport
  Attitude : Inport  Port=2
  Add : Sum  Inputs=+-
  Add1 : Sum
  Add2 : Sum
  Constant : Constant
  Constant1 : Constant  Value=0
  Gain : Gain  Gain=64.94
  Gain1 : Gain  Gain=217.38
  If : If  IfExpression=u1<50  ElseIfExpressions=u1>=50  ShowElse=off
  If Action Subsystem : Subsystem  TreatAsAtomicUnit=on
  If Action Subsystem1 : Subsystem  TreatAsAtomicUnit=on
  If Action Subsystem2 : Subsystem  TreatAsAtomicUnit=on
  If Action Subsystem3 : Subsystem  TreatAsAtomicUnit=on
  If1 : If  IfExpression=u1<50  ElseIfExpressions=u1>=50  ShowElse=off
  Mux : Mux  Inputs=2
  Mux1 : Mux  Inputs=2
  Mux4 : Mux  Inputs=5
  Thrust Tidle : Interpolation_n-D  Table=|  InternalRulePriority=Speed
      | [1060	670	880	1140	1500	1860
      | 635	425	690	1010	1330	1700
      | 60	25	345	755	1130	1525
      | -1020	-710	-300	350	910	1360
      | -2700	-1900	-1300	-247	600	1100
      | -3600	-1400	-595	-342	-200	700]
  Thrust Tmax : Interpolation_n-D  Table=reshape([20000,21420,22700,24240,26070,28886,15000,15700,16860,18910,21075,23319,10800,11225,12250,13760,15975,18300,7000,7323,8154,9285,11115,13484,4000,4435,5000,5700,6860,8642,2500,2600,2835,3215,3950,5057],6,6)  InternalRulePriority=Speed
  Thrust Tmil : Interpolation_n-D  Table=|  InternalRulePriority=Speed
      | [12680	9150	6200	3950	2450	1400
      | 12680	9150	6313	4040	2470	1400
      | 12610	9312	6610	4290	2600	1560
      | 12640	9839	7090	4660	2840	1660
      | 12390	10176	7750	5320	3250	1930
      | 11680	9848	8050	6100	3800	2310]
  To Workspace : ToWorkspace  VariableName=T_max_min  SaveFormat=Timeseries  SampleTime=-1
  To Workspace1 : ToWorkspace  VariableName=check_engine  SaveFormat=Timeseries  SampleTime=-1
  To Workspace2 : ToWorkspace  VariableName=Mach_alt_input  SaveFormat=Timeseries  SampleTime=-1
  attitude Prelookup : PreLookup  BreakpointsData=[0,10000,20000,30000,40000,50000]  IndexSearchMethod=Linear search  BeginIndexSearchUsingPreviousIndexResult=on  DiagnosticForOutOfRangeInput=Warning
  constant : Constant  Value=117.38
  mach Prelookup : PreLookup  BreakpointsData=[0,0.2,0.4,0.6,0.8,1]  IndexSearchMethod=Linear search  BeginIndexSearchUsingPreviousIndexResult=on  DiagnosticForOutOfRangeInput=Warning
  T_max : Outport  VectorParamsAs1DForOutWhenUnconnected=off
  T_min : Outport  Port=2  VectorParamsAs1DForOutWhenUnconnected=off
  wires:
  Mach/1 -> Mux/2, mach Prelookup/1
  Attitude/1 -> attitude Prelookup/1, Mux/1
  Add2/1 -> T_min/1, Mux1/2
  Add1/1 -> T_max/1, Mux1/1
  attitude Prelookup/2 -> Thrust Tidle/4, Thrust Tmil/4, Thrust Tmax/4
  Mux1/1 -> To Workspace/1
  Thrust Tmil/1 -> Mux4/4
  Mux/1 -> To Workspace2/1
  Gain1/1 -> Add/1
  If Action Subsystem1/1(T_max1) -> Add1/2
  Constant/1 -> Gain1/1
  mach Prelookup/1 -> Thrust Tidle/1, Thrust Tmil/1, Thrust Tmax/1
  If/2 -> If Action Subsystem1/Action
  If1/2 -> If Action Subsystem3/Action
  If Action Subsystem3/1(T_min) -> Add2/2
  If Action Subsystem2/1(T_min) -> Add2/1
  If1/1 -> If Action Subsystem2/Action
  Gain/1 -> Mux4/2, If1/1
  If Action Subsystem/1(T_max1) -> Add1/1
  Thrust Tmax/1 -> Mux4/5
  mach Prelookup/2 -> Thrust Tidle/2, Thrust Tmil/2, Thrust Tmax/2
  Thrust Tidle/1 -> Mux4/3
  If/1 -> If Action Subsystem/Action
  Add/1 -> Mux4/1, If/1
  constant/1 -> Add/2
  Mux4/1 -> If Action Subsystem1/1("input "), If Action Subsystem2/1("input "), If Action Subsystem3/1("input "), To Workspace1/1, If Action Subsystem/1("input ")
  Constant1/1 -> Gain/1
  attitude Prelookup/1 -> Thrust Tidle/3, Thrust Tmil/3, Thrust Tmax/3

== system example_main_NDI_f16/F-16 Vehicle Systems Model/Vehicle/Aerodynamics/Aerofynamic Coefficients ==
  note: Total Velocity
  note: 未建模，缺少數據
  note: speed brake
      | 減速板
  note: leading-edge flaps
      | 前緣襟翼
  alpha (deg) : Inport
  beta (deg) : Inport  Port=2
  LEF (deg) : Inport  Port=3
  elevator (deg) : Inport  Port=4
  alieron (deg) : Inport  Port=5
  rudder (deg) : Inport  Port=6
  SB (deg) : Inport  Port=7
  vt (ft/s) : Inport  Port=8
  p : Inport  Port=9
  q : Inport  Port=10
  r : Inport  Port=11
  GearAngle : Inport  Port=12
  h_AGL : Inport  Port=13
  Add : Sum  Inputs=+-
  CXT : Subsystem
  CYT : Subsystem
  CZT : Subsystem
  ClT : Subsystem
  CmT : Subsystem
  CnT : Subsystem
  Constant3 : Constant
  Divide2 : Product  Inputs=**/
  Divide3 : Product  Inputs=**/
  Divide4 : Product  Inputs=**/
  Gain1 : Gain  Gain=2
  Ground Effects : Subsystem  Commented=on
  Landing Gear Effects : Subsystem  Commented=on
  Terminator : Terminator  Commented=on
  Terminator1 : Terminator  Commented=on
  b(ft) : Constant  Value=ac.b
  cbar(ft) : Constant  Value=ac.cbar
  center of gravity as a fraction of cbar : Constant  Value=ac.x_cg
  r2d1 : Gain  Gain=1/25  SaturateOnIntegerOverflow=on  OutDataTypeStr=Inherit: Same as input  ParamDataTypeStr=Inherit: Same as input
  r2d2 : Gain  Gain=1/20  SaturateOnIntegerOverflow=on  OutDataTypeStr=Inherit: Same as input  ParamDataTypeStr=Inherit: Same as input
  r2d3 : Gain  Gain=1/60  SaturateOnIntegerOverflow=on  OutDataTypeStr=Inherit: Same as input  ParamDataTypeStr=Inherit: Same as input
  r2d4 : Gain  Gain=1/30  SaturateOnIntegerOverflow=on  OutDataTypeStr=Inherit: Same as input  ParamDataTypeStr=Inherit: Same as input
  reference center of gravity as a fraction of cbar : Constant  Value=ac.x_cg_ref
  CX_T : Outport  VectorParamsAs1DForOutWhenUnconnected=off
  CY_T : Outport  Port=2  VectorParamsAs1DForOutWhenUnconnected=off
  CZ_T : Outport  Port=3  VectorParamsAs1DForOutWhenUnconnected=off
  Cl_T : Outport  Port=4  VectorParamsAs1DForOutWhenUnconnected=off
  Cm_T : Outport  Port=5  VectorParamsAs1DForOutWhenUnconnected=off
  Cn_T : Outport  Port=6  VectorParamsAs1DForOutWhenUnconnected=off
  wires:
  alpha (deg)/1 -> ClT/1(alpha (deg)), CnT/1(alpha (deg)), CmT/1(alpha (deg)), CZT/1(alpha (deg)), CYT/1(alpha (deg)), CXT/1(alpha (deg))  "alpha"
  beta (deg)/1 -> ClT/2(beta (deg)), CnT/2(beta (deg)), CmT/2(beta (deg)), CZT/2(beta (deg)), CYT/2(beta (deg)), CXT/2("beta (deg) ")  "beta"
  elevator (deg)/1 -> ClT/3(elevator (deg)), CnT/3(elevator (deg)), CmT/3(elevator (deg)), CZT/3(elevator (deg)), CXT/3(elevator (deg))  "elevator"
  vt (ft/s)/1 -> Gain1/1
  q/1 -> Divide2/1  "q"
  r/1 -> Divide3/1  "r"
  Divide2/1 -> CXT/5(qc_2v), CZT/5(qc_2v), CmT/5(qc_2v)  "qc_2v"
  Divide3/1 -> CYT/6(rb_2v), ClT/7(rb_2v), CnT/7(rb_2v)  "rb_2v"
  Divide4/1 -> CYT/7(pb_2v), ClT/8(pb_2v), CnT/8(pb_2v)  "pb_2v"
  b(ft)/1 -> CnT/12(b), Divide3/2, Divide4/2  "b"
  cbar(ft)/1 -> CnT/11(cbar), Divide2/2  "cbar"
  reference center of gravity as a fraction of cbar/1 -> CmT/6(x_cg_ref), CnT/9(x_cg_ref)
  center of gravity as a fraction of cbar/1 -> CmT/7(x_cg), CnT/10(x_cg)
  CZT/1(Cz_tot) -> CmT/8(Cz_tot), CZ_T/1
  CYT/1(Cy_tot) -> CnT/13(Cy_tot), CY_T/1
  CXT/1(Cx_tot) -> CX_T/1
  ClT/1(Cl_tot) -> Cl_T/1
  CmT/1(Cm_tot) -> Cm_T/1
  CnT/1(Cn_tot) -> Cn_T/1
  Add/1 -> CmT/4(dlef), CnT/6(dlef), ClT/6(dlef), CZT/4(dlef), CYT/3(dlef), CXT/4(dlef)  "dlef"
  alieron (deg)/1 -> r2d2/1
  rudder (deg)/1 -> r2d4/1
  SB (deg)/1 -> r2d3/1
  r2d1/1 -> Add/2
  Constant3/1 -> Add/1
  LEF (deg)/1 -> r2d1/1
  Gain1/1 -> Divide4/3, Divide3/3, Divide2/3  "2v"
  p/1 -> Divide4/1  "p"
  r2d3/1 -> CZT/6(sb), CmT/9(sb), CXT/6(sb)
  r2d2/1 -> CnT/4(dail), ClT/5(dail), CYT/4(dail)
  r2d4/1 -> CYT/5(drud), CnT/5(drud), ClT/4(drud)
  GearAngle/1 -> Landing Gear Effects/3(Landing Gear Angle)
  h_AGL/1 -> Ground Effects/3(h_AGL)
  Landing Gear Effects/1(Coeff) -> Terminator/1
  Ground Effects/1(Coeff) -> Terminator1/1
